simulink subsystem "LinearPendulum"  (R2025b)
settings: Solver=VariableStepAuto  StartTime=0.0  StopTime=10.0  RelTol=1e-3
model mask{b=0.86, g=9.81, l=0.1, phi0=pi/4, dphi0=0}
  mask prompts: b "Friction Coefficient"; g "Gravity"; l "Rod Length"; phi0 "Initial Position"; dphi0 "Initial Velocity"
settings Model: Creator=alvaro  LastModifiedBy=alvaro

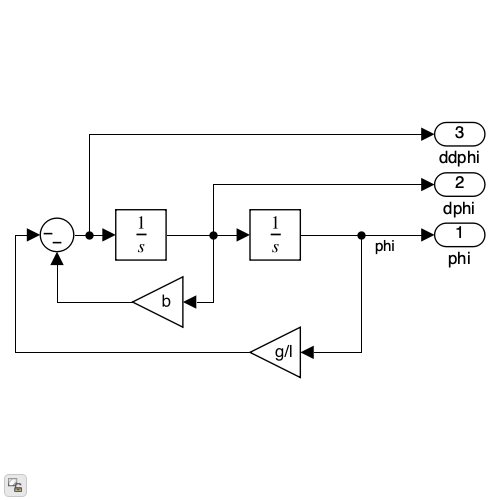
[thumbnail: Simulink's stored preview of the top-level diagram]
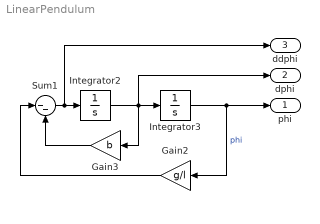
== system LinearPendulum ==
  Gain2 : Gain  Gain=g/l
  Gain3 : Gain  Gain=b
  Integrator2 : Integrator  InitialCondition=dphi0
  Integrator3 : Integrator  InitialCondition=phi0
  Sum1 : Sum  Inputs=|--
  phi : Outport
  dphi : Outport  Port=2
  ddphi : Outport  Port=3
  wires:
  Gain2/1 -> Sum1/1
  Gain3/1 -> Sum1/2
  Integrator3/1 -> Gain2/1, phi/1  "phi"
  Sum1/1 -> Integrator2/1, ddphi/1
  Integrator2/1 -> Integrator3/1, Gain3/1, dphi/1
